simulink model "BaseEngineController_LS"  (Simulink 7.7)
settings: Solver=FixedStepDiscrete  StartTime=0.0  StopTime=10.0  RelTol=1e-3
PreLoadFcn:
  | try, eval([bdroot '_setup']); catch, eval('model_setup', ''); end
InitFcn:
  | try, eval([bdroot '_setup']); catch, eval('model_setup', ''); end
undefined symbols (not defined in the file): ECU555, High, motohawk_build_version, motohawk_trunc_name, motohawk_vardec_config_group, motohawk_vardec_path, True
libraries: MotoHawk_lib x1418, motohawk_control_primitives_lib x183, motohawk_engine_lib x32, simulink x21, motohawk_annotations_lib x9, AutoDoc_lib x8, simulink_extras x4, motohawk_ccp_examples_lib x1, motohawk_control_primitives_motoshare_lib x1
(part 21 of 27)

== system BaseEngineController_LS/Foreground/Control/Controller/Run/Fuel System Manager/O2 Fuel Adapt ==
  O2 Info : Inport
  Sensors : Inport  Port=2
  Abs : Abs  SaturateOnIntegerOverflow=on
  Adapt FuelFlowComp Map Bank A : Subsystem  TreatAsAtomicUnit=on
  Adapt FuelFlowComp Map Bank B : Subsystem  TreatAsAtomicUnit=on
  Bus Selector1 : BusSelector  OutputSignals=O2Error.O2ITerm_BankA
  Bus Selector2 : BusSelector  OutputSignals=O2ControlEnable.BankAEnable
  Bus Selector3 : BusSelector  OutputSignals=RawIndexes.MAP09Idx,RawIndexes.RPM09Idx
  Bus Selector4 : BusSelector  OutputSignals=DesiredLambda.WarmUpRatio,DesiredLambda.WarmUptimeRatio,DesiredLambda.DesEquivRatio
  Bus Selector5 : BusSelector  OutputSignals=O2Error.O2ITerm_BankB
  Divide : Product  Inputs=**
  Divide1 : Product  Inputs=**
  Logical Operator2 : Logic  Inputs=5
  MinMax : MinMax  Function=max  Inputs=2
  O2 Control Enable Delay : Subsystem  TreatAsAtomicUnit=on
  Product0 : Product  SaturateOnIntegerOverflow=on  InputSameDT=on  OutDataTypeStr=Inherit: Same as first input
  Product1 : Product  SaturateOnIntegerOverflow=on  InputSameDT=on  OutDataTypeStr=Inherit: Same as first input
  Relational Operator : RelationalOperator  Operator=<=  InputSameDT=on
  Saturation (Tunable) : Subsystem  AncestorBlock=motohawk_control_primitives_lib/Saturation (Tunable)  mask(Saturation (Tunable)){prefix='FuelAdaptError_BankA', UprLim=1, LwrLim=-1, units='', grp=motohawk_vardec_path(gcb)}
      mask prompts: UprLim "Upper Limit"; LwrLim "Lower Limit"; grp "MotoTune Group String"
      mask help: Saturation block with calibratable min/max values.
      mask Display:
      | patch([0 0 1 1], [0 0.075 0.075 0], [230/255 0/255 0/255])
      | patch([0 0 1 1], [0.025 0.05 0.05 0.025], [150/255 0/255 0/255])
      | patch([0 0 1 1], [0 0.025 0.025 0], [0/255 0/255 0/255])
      | 
      | plot([0 .2 .8 1], [.1 .1 1 1])
  Saturation (Tunable)1 : Subsystem  AncestorBlock=motohawk_control_primitives_lib/Saturation (Tunable)  mask(Saturation (Tunable)){prefix='FuelAdaptError_BankB', UprLim=1, LwrLim=-1, units='', grp=motohawk_vardec_path(gcb)}
      mask prompts: UprLim "Upper Limit"; LwrLim "Lower Limit"; grp "MotoTune Group String"
      mask help: Saturation block with calibratable min/max values.
      mask Display:
      | patch([0 0 1 1], [0 0.075 0.075 0], [230/255 0/255 0/255])
      | patch([0 0 1 1], [0.025 0.05 0.05 0.025], [150/255 0/255 0/255])
      | patch([0 0 1 1], [0 0.025 0.025 0], [0/255 0/255 0/255])
      | 
      | plot([0 .2 .8 1], [.1 .1 1 1])
  WarmUp Disable : Subsystem  TreatAsAtomicUnit=on
  motohawk_calibration : MotoHawk_lib/Calibration & Probing Blocks/motohawk_calibration  nam='AdaptEnable'  val=true  storage=Calibration  show_more=on  name_source=Use Parameter  data_type=Inherit from 'Default Value'  read_level=1  write_level=1  ovr_cals=on  view_as=Enumeration  enum_struct={'Disabled', 'Enabled'}  vector_style=Wide Row  use_help_units=on  help='Determines whether the FuelFlowComp map will be adapted using the MAF sensor'  units='bool'  use_header_enum=off  row_header_enum={}  col_header_enum={}  use_min_max=off  min_val=-inf  max_val=inf  use_precision=off  precision=''  gain=1  offset=0  exp=1  use_mototune_group=on  mototune_group=motohawk_vardec_path(gcb)
  motohawk_calibration1 : MotoHawk_lib/Calibration & Probing Blocks/motohawk_calibration  nam='FuelAdaptDelta'  val=0.5  storage=Calibration  show_more=on  name_source=Use Parameter  data_type=Inherit from 'Default Value'  read_level=1  write_level=1  ovr_cals=on  view_as=Number  enum_struct={'Disabled', 'Enabled'}  vector_style=Wide Row  use_help_units=on  help='O2_Error must be less than this delta to adapt the FuelFlowComp map'  units='mult'  use_header_enum=off  row_header_enum={}  col_header_enum={}  use_min_max=on  min_val=0  max_val=2  use_precision=off  precision=''  gain=1  offset=0  exp=1  use_mototune_group=on  mototune_group=motohawk_vardec_path(gcb)
  motohawk_calibration2 : MotoHawk_lib/Calibration & Probing Blocks/motohawk_calibration  nam='FuelAdaptEnable'  val=false  storage=Calibration  show_more=on  name_source=Use Parameter  data_type=Inherit from 'Default Value'  read_level=1  write_level=1  ovr_cals=on  view_as=Enumeration  enum_struct={'Disabled', 'Enabled'}  vector_style=Wide Row  use_help_units=on  help='Determines whether the FuelFlowComp map will be adapted using the MAF sensor'  units='bool'  use_header_enum=off  row_header_enum={}  col_header_enum={}  use_min_max=off  min_val=-inf  max_val=inf  use_precision=off  precision=''  gain=1  offset=0  exp=1  use_mototune_group=on  mototune_group=motohawk_vardec_path(gcb)
  motohawk_interpolation_1d1 : MotoHawk_lib/Lookup Tables/motohawk_interpolation_1d  nam='FuelAdaptGain_BankA'  table_data=[0,0,0,0,0]  show_more=on  data_type=Inherit from 'Table Data'  storage=NonAdaptive  read_level=1  write_level=1  ovr_cals=on  use_help=on  help="'Gain for updating FuelFlowComp map.  This fraction of the error is added to the map every 5ms.'"  units=''  use_min_max=off  min_val=-inf  max_val=inf  use_precision=on  precision='1.4'  gain=1  offset=0  exp=1  use_links=off  prelookup_block=''  output_name=''  use_mototune_group=on  mototune_group=motohawk_vardec_path(gcb)
  motohawk_interpolation_1d2 : MotoHawk_lib/Lookup Tables/motohawk_interpolation_1d  nam='FuelAdaptGain_BankB'  table_data=[0,0,0,0,0]  show_more=on  data_type=Inherit from 'Table Data'  storage=NonAdaptive  read_level=1  write_level=1  ovr_cals=on  use_help=on  help="'Gain for updating FuelFlowComp map.  This fraction of the error is added to the map every 5ms.'"  units=''  use_min_max=off  min_val=-inf  max_val=inf  use_precision=on  precision='1.4'  gain=1  offset=0  exp=1  use_links=off  prelookup_block=''  output_name=''  use_mototune_group=on  mototune_group=motohawk_vardec_path(gcb)
  motohawk_interpolation_2d1 : MotoHawk_lib/Lookup Tables/motohawk_interpolation_2d  nam='FuelFlowComp'  table_data=ones(9)  show_more=on  data_type=Inherit from 'Table Data'  storage=NonAdaptive  read_level=1  write_level=1  ovr_cals=on  use_help=on  help='Fuel Flow Compensation Multiplier - gain to adjust modelling errors in mechanical fuel system.'  units='mult'  use_min_max=on  min_val=-inf  max_val=inf  use_precision=on  precision=''  gain=1  offset=0  exp=1  use_links=off  row_prelookup_block=''  col_prelookup_block=''  output_name=''  use_mototune_group=on  mototune_group=motohawk_vardec_path(gcb)
  motohawk_interpolation_2d2 : MotoHawk_lib/Lookup Tables/motohawk_interpolation_2d  nam='FuelFlowCompAdapt_BankA'  table_data=ones(9)  show_more=on  data_type=Inherit from 'Table Data'  storage=Adaptive - NonVolatile  read_level=1  write_level=1  ovr_cals=on  use_help=on  help='Adapt map based on O2 ITerm that is multiplied into FuelFlowComp.'  units='mult'  use_min_max=on  min_val=-inf  max_val=inf  use_precision=on  precision=''  gain=1  offset=0  exp=1  use_links=off  row_prelookup_block=''  col_prelookup_block=''  output_name=''  use_mototune_group=on  mototune_group=motohawk_vardec_path(gcb)
  motohawk_interpolation_2d3 : MotoHawk_lib/Lookup Tables/motohawk_interpolation_2d  nam='FuelFlowCompAdapt_BankB'  table_data=ones(9)  show_more=on  data_type=Inherit from 'Table Data'  storage=Adaptive - NonVolatile  read_level=1  write_level=1  ovr_cals=on  use_help=on  help='Adapt map based on O2 ITerm that is multiplied into FuelFlowComp.'  units='mult'  use_min_max=on  min_val=-inf  max_val=inf  use_precision=on  precision=''  gain=1  offset=0  exp=1  use_links=off  row_prelookup_block=''  col_prelookup_block=''  output_name=''  use_mototune_group=on  mototune_group=motohawk_vardec_path(gcb)
  motohawk_prelookup1 : MotoHawk_lib/Lookup Tables/motohawk_prelookup  nam='O2ITerm_BankB'  breakpoint_data=[0,0,0,0,0]  show_more=on  data_type=Inherit from 'Table Data'  storage=Constant  read_level=1  write_level=1  ovr_cals=on  use_help=on  help='Index for O2 ITerm.'  units='mult'  use_min_max=off  min_val=-inf  max_val=inf  use_precision=off  precision=''  gain=1  offset=0  exp=1  use_links=on  input_name=''  use_mototune_group=on  mototune_group=motohawk_vardec_path(gcb)
  motohawk_prelookup13 : MotoHawk_lib/Lookup Tables/motohawk_prelookup  nam='O2ITerm_BankA'  breakpoint_data=[0,0,0,0,0]  show_more=on  data_type=Inherit from 'Table Data'  storage=Constant  read_level=1  write_level=1  ovr_cals=on  use_help=on  help='Index for O2 ITerm.'  units='mult'  use_min_max=off  min_val=-inf  max_val=inf  use_precision=off  precision=''  gain=1  offset=0  exp=1  use_links=on  input_name=''  use_mototune_group=on  mototune_group=motohawk_vardec_path(gcb)
  motohawk_probe1 : MotoHawk_lib/Calibration & Probing Blocks/motohawk_probe  nam='FuelAdapt_Error_BankB'  show_more=on  name_source=Use Parameter  read_level=1  view_as=Number  enum_struct={'Disabled', 'Enabled'}  vector_style=Wide Row  use_help_units=on  help='Error in fuel flow at the current operating point, as compared to O2 sensor'  units=''  use_header_enum=off  row_header_enum={}  col_header_enum={}  use_precision=off  precision=''  gain=1  offset=0  exp=1  use_mototune_group=on  mototune_group=motohawk_vardec_path(gcb)
  motohawk_probe3 : MotoHawk_lib/Calibration & Probing Blocks/motohawk_probe  nam='FuelAdaptEnabled'  show_more=on  name_source=Use Parameter  read_level=1  view_as=Enumeration  enum_struct={'Not Enabled', 'Enabled'}  vector_style=Wide Row  use_help_units=on  help='Indicates whether FuelFlowComp map adapting is enabled'  units=''  use_header_enum=off  row_header_enum={}  col_header_enum={}  use_precision=off  precision=''  gain=1  offset=0  exp=1  use_mototune_group=on  mototune_group=motohawk_vardec_path(gcb)
  motohawk_probe7 : MotoHawk_lib/Calibration & Probing Blocks/motohawk_probe  nam='FuelAdapt_Error_BankA'  show_more=on  name_source=Use Parameter  read_level=1  view_as=Number  enum_struct={'Disabled', 'Enabled'}  vector_style=Wide Row  use_help_units=on  help='Error in fuel flow at the current operating point, as compared to O2 sensor'  units=''  use_header_enum=off  row_header_enum={}  col_header_enum={}  use_precision=off  precision=''  gain=1  offset=0  exp=1  use_mototune_group=on  mototune_group=motohawk_vardec_path(gcb)
  "Adapt Fuel Mult Bank A " : Outport
  Adapt Fuel Mult Bank B : Outport  Port=2
  wires:
  Abs/1 -> Relational Operator/1
  motohawk_calibration1/1 -> Relational Operator/2
  motohawk_interpolation_1d1/1 -> Product0/2
  Product0/1 -> Saturation (Tunable)/1(In)
  Sensors/1 -> Bus Selector3/1
  O2 Info/1 -> Bus Selector2/1, Bus Selector4/1, Bus Selector1/1, Bus Selector5/1
  Bus Selector1/1 -> motohawk_prelookup13/1, Product0/1, MinMax/1  "<O2ITerm_BankA>"
  Bus Selector2/1 -> O2 Control Enable Delay/1(State_In)  "<BankAEnable>"
  Relational Operator/1 -> Logical Operator2/5
  WarmUp Disable/1(State_Out) -> Logical Operator2/3
  O2 Control Enable Delay/1(State_Out) -> Logical Operator2/4
  Logical Operator2/1 -> Adapt FuelFlowComp Map Bank A/Enable, motohawk_probe3/1, Adapt FuelFlowComp Map Bank B/Enable
  Saturation (Tunable)/1(Out) -> Adapt FuelFlowComp Map Bank A/1(AdaptError), motohawk_probe7/1
  motohawk_calibration/1 -> Logical Operator2/2
  motohawk_calibration2/1 -> Logical Operator2/1
  motohawk_interpolation_2d1/1 -> Divide/1, Divide1/2
  Divide/1 -> "Adapt Fuel Mult Bank A "/1
  motohawk_interpolation_2d2/1 -> Adapt FuelFlowComp Map Bank A/2(Adapt), Divide/2
  Bus Selector3/1 -> motohawk_interpolation_2d2/1, motohawk_interpolation_2d1/1, motohawk_interpolation_2d3/1  "<MAP09Idx>"
  Bus Selector3/2 -> motohawk_interpolation_2d2/2, motohawk_interpolation_2d1/2, motohawk_interpolation_2d3/2  "<RPM09Idx>"
  Bus Selector4/3 -> WarmUp Disable/3(BaseRatio)  "<DesEquivRatio>"
  Bus Selector4/2 -> WarmUp Disable/2(WarmupTimeRatio)  "<WarmUptimeRatio>"
  Bus Selector4/1 -> WarmUp Disable/1(WarmupRatio)  "<WarmUpRatio>"
  motohawk_prelookup13/1 -> motohawk_interpolation_1d1/1
  motohawk_prelookup1/1 -> motohawk_interpolation_1d2/1
  Product1/1 -> Saturation (Tunable)1/1(In)
  Saturation (Tunable)1/1(Out) -> Adapt FuelFlowComp Map Bank B/1(AdaptError), motohawk_probe1/1
  motohawk_interpolation_1d2/1 -> Product1/2
  Bus Selector5/1 -> motohawk_prelookup1/1, Product1/1, MinMax/2  "<O2ITerm_BankB>"
  motohawk_interpolation_2d3/1 -> Divide1/1, Adapt FuelFlowComp Map Bank B/2(Adapt)
  Divide1/1 -> Adapt Fuel Mult Bank B/1
  MinMax/1 -> Abs/1

== system BaseEngineController_LS/Foreground/Control/Controller/Run/MaxGovernor/I-Term Preload ==
  TotalETCReq : Inport
  RPMAccelIdx : Inport  Port=2
  Sum : Sum  Inputs=|+-
  motohawk_interpolation_1d4 : MotoHawk_lib/Lookup Tables/motohawk_interpolation_1d  nam='MaxGovPreloadITerm'  table_data=[1 30 50 51.18 52.349998 53.529999 54.709999 55.880001 57.060001 58.240002 59.41 60.59 61.759998 62.939999 67.650002 68.82 70]  show_more=on  data_type=Inherit from 'Table Data'  storage=NonAdaptive  read_level=1  write_level=1  ovr_cals=on  use_help=on  help='Preload for Max Gov PID ITerm based on engine acceleration rate upon entry into max gov.'  units='%'  use_min_max=on  min_val=-inf  max_val=inf  use_precision=on  precision=''  gain=1  offset=0  exp=1  use_links=off  prelookup_block=''  output_name=''  use_mototune_group=on  mototune_group=motohawk_vardec_path(gcb)
  motohawk_probe : MotoHawk_lib/Calibration & Probing Blocks/motohawk_probe  nam='MaxGovIC'  show_more=on  name_source=Use Parameter  read_level=1  view_as=Number  enum_struct={'Disabled', 'Enabled'}  vector_style=Wide Row  use_help_units=off  help=''  units=''  use_header_enum=off  row_header_enum={}  col_header_enum={}  use_precision=off  precision=''  gain=1  offset=0  exp=1  use_mototune_group=on  mototune_group=motohawk_vardec_path(gcb)
  ITerm Preload : Outport
  wires:
  RPMAccelIdx/1 -> motohawk_interpolation_1d4/1
  Sum/1 -> ITerm Preload/1, motohawk_probe/1
  motohawk_interpolation_1d4/1 -> Sum/2
  TotalETCReq/1 -> Sum/1

== system BaseEngineController_LS/Foreground/Control/Controller/Run/MaxGovernor/MaxGovState ==
  note: Move into On State if RPM > EntryCriteria or Target.
      | Move into Trans State if APP falls below TPS, PID controller is frozen during Trans State, but output is based on APP.
      | 	When in AllSpeedGov mode, switch to Trans if AllSpeedGov setpoint is less than MaxGov setpoint minus hyst.
      | Move from Trans State back to On State if RPM > Target.
      | Move from Trans State to Off if RPM < Entry Criteria.
  RPMEntryCriteria : Inport
  TotalETCReq : Inport  Port=2
  Sensors : Inport  Port=3
  TargetRPM : Inport  Port=4
  Bus Selector : BusSelector  OutputSignals=RawProcessed.TPS
  Bus Selector1 : BusSelector  OutputSignals=Raw.RPMInst
  Constant : Constant  Value=boolean(0)
  Data Type Conversion : DataTypeConversion  OutDataTypeStr=int8
  Data Type Conversion1 : DataTypeConversion  OutDataTypeStr=int8
  Data Type Conversion2 : DataTypeConversion  OutDataTypeStr=int8
  Logical Operator : Logic  Operator=NOT  AllPortsSameDT=off  OutDataTypeStr=boolean
  Logical Operator1 : Logic  AllPortsSameDT=off  OutDataTypeStr=boolean
  Logical Operator2 : Logic  Operator=OR  AllPortsSameDT=off  OutDataTypeStr=boolean
  Logical Operator3 : Logic  Operator=OR  AllPortsSameDT=off  OutDataTypeStr=boolean
  MaxGOV Stateflow : Stateflow chart  TreatAsAtomicUnit=on
  Multiport Switch : MultiPortSwitch  DataPortOrder=Zero-based contiguous  Inputs=2  zeroidx=on
  Relational Operator : RelationalOperator  Operator=<=  OutDataTypeStr=boolean
  Relational Operator1 : RelationalOperator  Operator=>  OutDataTypeStr=boolean
  Relational Operator2 : RelationalOperator  Operator=>  OutDataTypeStr=boolean
  Sum : Sum  Inputs=|+-
  Sum1 : Sum  Inputs=++|
  motohawk_calibration1 : MotoHawk_lib/Calibration & Probing Blocks/motohawk_calibration  nam='MaxGovDisable'  val=0  storage=Calibration  show_more=on  name_source=Use Parameter  data_type=boolean  read_level=1  write_level=1  ovr_cals=on  view_as=Enumeration  enum_struct={'Gov Enabled', 'Gov Disabled'}  vector_style=Wide Row  use_help_units=on  help='Max governor manual disable'  units=''  use_header_enum=off  row_header_enum={}  col_header_enum={}  use_min_max=off  min_val=0  max_val=inf  use_precision=off  precision=''  gain=1  offset=0  exp=1  use_mototune_group=on  mototune_group=motohawk_vardec_path(gcb)
  motohawk_calibration5 : MotoHawk_lib/Calibration & Probing Blocks/motohawk_calibration  nam='MaxGovTPSHyst'  val=4  storage=Calibration  show_more=on  name_source=Use Parameter  data_type=Inherit from 'Default Value'  read_level=1  write_level=1  ovr_cals=on  view_as=Number  enum_struct={'Disabled', 'Enabled'}  vector_style=Wide Row  use_help_units=on  help='Hysterisis around max gov TPS entry criteria.'  units='%'  use_header_enum=off  row_header_enum={}  col_header_enum={}  use_min_max=on  min_val=0  max_val=inf  use_precision=on  precision=''  gain=1  offset=0  exp=1  use_mototune_group=on  mototune_group=motohawk_vardec_path(gcb)
  motohawk_data_def : MotoHawk_lib/Data Storage Blocks/motohawk_data_def  nam='MaxGov'  container_nam=''  data=0  typ=double  struct_nam='MyStruct'  storage=Volatile  outputRef=off  use_vardec=off  window=Display  read_level=1  write_level=1  ovr_cals=on  view_as=Number  enum_struct={'Disabled', 'Enabled'}  vector_style=Wide Row  use_help_units=off  help=''  units=''  use_header_enum=off  row_header_enum=''  col_header_enum=''  use_min_max=off  min_val=-inf  max_val=inf  use_precision=off  precision=''  gain=1  offset=0  exp=1  use_mototune_group=off  mototune_group=motohawk_vardec_path(gcb)  eval_name=MyData  data_stores=motohawk_sfun_data_def_data_stores  struct_instances=motohawk_sfun_data_def_struct_instances  vardecs=motohawk_sfun_data_def_vardecs
  motohawk_data_read : MotoHawk_lib/Data Storage Blocks/motohawk_data_read  source=Lookup By Name  structure=Scalar  operation=Read scalar from location by index  sz_vec=4  sz_row=2  sz_col=3  typ=double  nam='MaxGov'  checkNull=on  struct_inst_name='MyData'  struct_nam='MyStruct'
  motohawk_data_write : MotoHawk_lib/Data Storage Blocks/motohawk_data_write  source=Lookup By Name  structure=Scalar  operation=Write entire data structure at once  sz_vec=9  sz_row=2  sz_col=9  typ=double  nam='MaxGov'  checkNull=on  write_read_only=off  struct_inst_name=''  struct_name='MyStruct'
  motohawk_probe : MotoHawk_lib/Calibration & Probing Blocks/motohawk_probe  nam='MaxGovETCMode'  show_more=on  name_source=Use Parameter  read_level=1  view_as=Enumeration  enum_struct={'ETC Req Mode','PID Mode'}  vector_style=Wide Row  use_help_units=on  help=''  units=''  use_header_enum=off  row_header_enum={}  col_header_enum={}  use_precision=on  precision=''  gain=1  offset=0  exp=1  use_mototune_group=on  mototune_group=motohawk_vardec_path(gcb)
  motohawk_probe1 : MotoHawk_lib/Calibration & Probing Blocks/motohawk_probe  nam='MaxGovHold'  show_more=on  name_source=Use Parameter  read_level=1  view_as=Enumeration  enum_struct={'Hold Off','Hold On'}  vector_style=Wide Row  use_help_units=on  help=''  units=''  use_header_enum=off  row_header_enum={}  col_header_enum={}  use_precision=on  precision=''  gain=1  offset=0  exp=1  use_mototune_group=on  mototune_group=motohawk_vardec_path(gcb)
  motohawk_probe2 : MotoHawk_lib/Calibration & Probing Blocks/motohawk_probe  nam='MaxGovReset'  show_more=on  name_source=Use Parameter  read_level=1  view_as=Enumeration  enum_struct={'Reset Off','Reset On'}  vector_style=Wide Row  use_help_units=on  help=''  units=''  use_header_enum=off  row_header_enum={}  col_header_enum={}  use_precision=on  precision=''  gain=1  offset=0  exp=1  use_mototune_group=on  mototune_group=motohawk_vardec_path(gcb)
  motohawk_probe4 : MotoHawk_lib/Calibration & Probing Blocks/motohawk_probe  nam='MaxGovState'  show_more=on  name_source=Use Parameter  read_level=1  view_as=Enumeration  enum_struct={'Disabled', 'Enabled'}  vector_style=Wide Row  use_help_units=off  help=''  units=''  use_header_enum=off  row_header_enum={}  col_header_enum={}  use_precision=off  precision=''  gain=1  offset=0  exp=1  use_mototune_group=on  mototune_group=motohawk_vardec_path(gcb)
  ETCMode : Outport
  PIDReset : Outport  Port=2
  PIDHold : Outport  Port=3
  wires:
  Relational Operator/1 -> MaxGOV Stateflow/2(OnToTrans)
  motohawk_calibration5/1 -> Sum/2, Sum1/1
  Sensors/1 -> Bus Selector/1, Bus Selector1/1
  Bus Selector/1 -> Sum/1, Sum1/2  "<TPS>"
  Sum/1 -> Relational Operator/2
  Sum1/1 -> Relational Operator1/2
  TotalETCReq/1 -> Relational Operator/1, Relational Operator1/1
  RPMEntryCriteria/1 -> Logical Operator1/1, Logical Operator/1, Logical Operator3/1
  Relational Operator1/1 -> Logical Operator1/2
  MaxGOV Stateflow/3(Hold) -> Data Type Conversion1/1
  Logical Operator/1 -> MaxGOV Stateflow/4(TransToOff)
  Bus Selector1/1 -> Relational Operator2/1  "<RPMInst>"
  TargetRPM/1 -> Relational Operator2/2
  Logical Operator2/1 -> MaxGOV Stateflow/3(TransToOn)
  Logical Operator1/1 -> Logical Operator2/1
  Relational Operator2/1 -> Logical Operator2/2, Logical Operator3/2
  MaxGOV Stateflow/2(Reset) -> Data Type Conversion/1
  Logical Operator3/1 -> MaxGOV Stateflow/1(OffToOn)
  MaxGOV Stateflow/1(ETCMode) -> Data Type Conversion2/1
  Multiport Switch/1 -> ETCMode/1, motohawk_probe4/1, motohawk_probe/1
  Constant/1 -> Multiport Switch/3
  MaxGOV Stateflow/4(StateO) -> motohawk_data_write/1
  motohawk_data_read/1 -> MaxGOV Stateflow/5(State)
  Data Type Conversion/1 -> PIDReset/1, motohawk_probe2/1
  Data Type Conversion1/1 -> PIDHold/1, motohawk_probe1/1
  Data Type Conversion2/1 -> Multiport Switch/2
  motohawk_calibration1/1 -> Multiport Switch/1

== system BaseEngineController_LS/Foreground/Control/Controller/Run/MaxGovernor/Ramp RPM ==
  note: 1st-Order Ramp Up
  note: y[k] = a*x[k] + (1-a)*y[k-1]
  note: where a = t/T
  OnIdle : Inport
  TargetRPM : Inport  Port=2
  RPM : Inport  Port=3
  Constant : Constant  OutDataTypeStr=Inherit: Inherit via back propagation
  Don't allow setpoint to ever go above the TargetRPM : MinMax  Inputs=2  SaturateOnIntegerOverflow=on  InputSameDT=on
  Logical Operator : Logic  Operator=NOT
  Preload lowpass filter with current RPM while not on Idle : Switch  Threshold=0.5  ZeroCross=off  SaturateOnIntegerOverflow=on  InputSameDT=on
  Product1 : Product  Inputs=*/  SaturateOnIntegerOverflow=on  InputSameDT=on  OutDataTypeStr=Inherit: Same as first input
  Product2 : Product  SaturateOnIntegerOverflow=on  InputSameDT=on  OutDataTypeStr=Inherit: Same as first input
  Product3 : Product  SaturateOnIntegerOverflow=on  InputSameDT=on  OutDataTypeStr=Inherit: Same as first input
  Sum : Sum  Inputs=-+|  SaturateOnIntegerOverflow=on
  Sum1 : Sum  SaturateOnIntegerOverflow=on
  Unit Delay : UnitDelay  SampleTime=-1
  motohawk_calibration2 : MotoHawk_lib/Calibration & Probing Blocks/motohawk_calibration  nam='MaxGovRPMCtrlEntryFiltC'  val=0.2  storage=Calibration  show_more=on  name_source=Use Parameter  data_type=Inherit from 'Default Value'  read_level=1  write_level=1  ovr_cals=on  view_as=Number  enum_struct={'Disabled', 'Enabled'}  vector_style=Wide Row  use_help_units=on  help='Filter rate at which Max Gov setup is increased to MaxGovBaseRPMSetpoint.'  units='sec'  use_header_enum=off  row_header_enum={}  col_header_enum={}  use_min_max=on  min_val=.005  max_val=inf  use_precision=off  precision=''  gain=1  offset=0  exp=1  use_mototune_group=on  mototune_group=motohawk_vardec_path(gcb)
  motohawk_delta_time : MotoHawk_lib/Extra Development Blocks/motohawk_delta_time  samp_time=-1  init_val=0  mode=Seconds (double)
  motohawk_probe3 : MotoHawk_lib/Calibration & Probing Blocks/motohawk_probe  nam='MaxGovRPMSetpoint'  show_more=on  name_source=Use Parameter  read_level=1  view_as=Number  enum_struct={'Disabled', 'Enabled'}  vector_style=Wide Row  use_help_units=on  help='RPMSetpoint of Max Gov controller.'  units='RPM'  use_header_enum=off  row_header_enum={}  col_header_enum={}  use_precision=on  precision=''  gain=1  offset=0  exp=1  use_mototune_group=on  mototune_group=motohawk_vardec_path(gcb)
  RPMSetPt : Outport
  wires:
  Logical Operator/1 -> Preload lowpass filter with current RPM while not on Idle/2
  Don't allow setpoint to ever go above the TargetRPM/1 -> RPMSetPt/1, Unit Delay/1, motohawk_probe3/1
  Preload lowpass filter with current RPM while not on Idle/1 -> Don't allow setpoint to ever go above the TargetRPM/2
  RPM/1 -> Preload lowpass filter with current RPM while not on Idle/1
  TargetRPM/1 -> Don't allow setpoint to ever go above the TargetRPM/1, Product2/1
  Product1/1 -> Sum/1, Product2/2  "alpha"
  Constant/1 -> Sum/2
  Product2/1 -> Sum1/1
  Product3/1 -> Sum1/2
  Sum/1 -> Product3/1
  Unit Delay/1 -> Product3/2
  motohawk_delta_time/1 -> Product1/1
  motohawk_calibration2/1 -> Product1/2
  Sum1/1 -> Preload lowpass filter with current RPM while not on Idle/3
  OnIdle/1 -> Logical Operator/1

== system BaseEngineController_LS/Foreground/Control/Controller/Run/MaxGovernor/Trigger Pre-load ==
  RPM : Inport
  GearState : Inport  Port=2
  InGear : Subsystem  TreatAsAtomicUnit=on
  InNeutral : Subsystem  TreatAsAtomicUnit=on
  Logical Operator : Logic  Operator=NOT  AllPortsSameDT=off  OutDataTypeStr=boolean
  Merge : Merge
  Merge1 : Merge
  Relational Operator : RelationalOperator  Operator=>  OutDataTypeStr=boolean
  Sum1 : Sum  Inputs=+-|
  Trigger : Outport
  BaseRPMSetpoint : Outport  Port=2
  wires:
  Relational Operator/1 -> Trigger/1
  RPM/1 -> Relational Operator/1
  Sum1/1 -> Relational Operator/2
  InGear/1(BaseSetpoint) -> Merge/1
  InGear/2(Threshold) -> Merge1/1
  InNeutral/1(BaseSetpoint) -> Merge/2
  InNeutral/2(Threshold) -> Merge1/2
  Merge/1 -> Sum1/1, BaseRPMSetpoint/1
  Merge1/1 -> Sum1/2
  GearState/1 -> InGear/Enable, Logical Operator/1
  Logical Operator/1 -> InNeutral/Enable

== system BaseEngineController_LS/Foreground/Control/Controller/Run/MaxGovernor/Universal PID (Tunable & Scheduled) ==
  ITerm IC : Inport
  Reset All : Inport  Port=2
  Hold PID : Inport  Port=3
  SetPoint : Inport  Port=4
  Actual : Inport  Port=5
  Constant : Constant  Value=0
  Product3 : Product  SaturateOnIntegerOverflow=on  InputSameDT=on  OutDataTypeStr=Inherit: Same as first input
  Product4 : Product  SaturateOnIntegerOverflow=on  InputSameDT=on  OutDataTypeStr=Inherit: Same as first input
  Product5 : Product  SaturateOnIntegerOverflow=on  InputSameDT=on  OutDataTypeStr=Inherit: Same as first input
  Saturation : motohawk_control_primitives_lib/Saturation  SystemSampleTime=-1
  Switch : Switch  Threshold=1
  Switch1 : Switch  Threshold=1
  Universal PID : motohawk_control_primitives_lib/Universal PID  Description=|  SystemSampleTime=-1  samp_time=.005
      | /* Name: ErrorGain Unit:mult ClassID:VAR StorageID:FLASH Access:RW4+RW3+NA2+NA1 TypeID:UINT4                   
      |    Gain:0.000000001 Min:0.000000000 Max:4.000000000 Format:10.9 UpdateID:REMOTE Help:"This gain is applied to "
      |    "the error term before it is used to calculate the P, I and D terms." VardecSig:6C */                       
      |                                                                                                                
      | /* Name: ITermLowerLim Unit:0 ClassID:VAR StorageID:FLASH Access:RW4+RW3+NA2+NA1 TypeID:SINT2 Gain:0.1         
      |    Min:-3276.8 Max:3276.7 Format:5.1 UpdateID:REMOTE Help:"Lower limit on the I-term value." VardecSig:6C */   
      |                                                                                                                
      | /* Name: ITermUpperLim ClassID:VAR StorageID:FLASH Access:RW4+RW3+NA2+NA1 TypeID:SINT2 Gain:0.1 Min:-3276.8    
      |    Max:3276.7 Format:5.1 UpdateID:REMOTE Help:"Upper limit on I-term value." VardecSig:6C */                   
      |                                                                                                                
      | /* Name: PIDOutLowerLim ClassID:VAR StorageID:FLASH Access:RW4+RW3+NA2+NA1 TypeID:SINT2 Gain:0.1               
      |    Min:-3276.8 Max:3276.7 Format:5.1 UpdateID:REMOTE Help:"Lower limit on PID output." VardecSig:6C */         
      |                                                                                                                
      | /* Name: PIDOutUpperLim ClassID:VAR StorageID:FLASH Access:RW4+RW3+NA2+NA1 TypeID:SINT2 Gain:0.1               
      |    Min:-3276.8 Max:3276.7 Format:3.1 UpdateID:REMOTE Help:"Upper limit on PID output." VardecSig:6C */
  motohawk_calibration2 : MotoHawk_lib/Calibration & Probing Blocks/motohawk_calibration  nam=[prefix 'PIDOutUpperLimit']  val=100  storage=Calibration  show_more=on  name_source=Use Parameter  data_type=Inherit from 'Default Value'  read_level=1  write_level=1  ovr_cals=on  view_as=Number  enum_struct={'Disabled', 'Enabled'}  vector_style=Wide Row  use_help_units=on  help='Upper limit on max governor PID Output.'  units='%'  use_header_enum=off  row_header_enum={}  col_header_enum={}  use_min_max=on  min_val=-inf  max_val=inf  use_precision=on  precision=''  gain=1  offset=0  exp=1  use_mototune_group=on  mototune_group=motohawk_vardec_path(gcb)
  motohawk_calibration3 : MotoHawk_lib/Calibration & Probing Blocks/motohawk_calibration  nam=[prefix 'PGain']  val=0.5  storage=Calibration  show_more=on  name_source=Use Parameter  data_type=Inherit from 'Default Value'  read_level=1  write_level=1  ovr_cals=on  view_as=Number  enum_struct={'Disabled', 'Enabled'}  vector_style=Wide Row  use_help_units=on  help='Base P-gain for the max. governor controller.'  units='mult'  use_header_enum=off  row_header_enum={}  col_header_enum={}  use_min_max=off  min_val=-inf  max_val=inf  use_precision=off  precision=''  gain=1  offset=0  exp=1  use_mototune_group=on  mototune_group=motohawk_vardec_path(gcb)
  motohawk_calibration4 : MotoHawk_lib/Calibration & Probing Blocks/motohawk_calibration  nam=[prefix 'IGain']  val=1  storage=Calibration  show_more=on  name_source=Use Parameter  data_type=Inherit from 'Default Value'  read_level=1  write_level=1  ovr_cals=on  view_as=Number  enum_struct={'Disabled', 'Enabled'}  vector_style=Wide Row  use_help_units=on  help='Base I-gain for the max. governor controller.'  units='mult'  use_header_enum=off  row_header_enum={}  col_header_enum={}  use_min_max=off  min_val=-inf  max_val=inf  use_precision=off  precision=''  gain=1  offset=0  exp=1  use_mototune_group=on  mototune_group=motohawk_vardec_path(gcb)
  motohawk_calibration5 : MotoHawk_lib/Calibration & Probing Blocks/motohawk_calibration  nam=[prefix 'ErrorGain']  val=0.1  storage=Calibration  show_more=on  name_source=Use Parameter  data_type=Inherit from 'Default Value'  read_level=1  write_level=1  ovr_cals=on  view_as=Number  enum_struct={'Disabled', 'Enabled'}  vector_style=Wide Row  use_help_units=on  help='Error gain for the max governor controller. This gain is applied to the RPM error term before it is used to calculate the P, I and D terms.'  units='mult'  use_header_enum=off  row_header_enum={}  col_header_enum={}  use_min_max=on  min_val=-inf  max_val=inf  use_precision=off  precision=''  gain=1  offset=0  exp=1  use_mototune_group=on  mototune_group=motohawk_vardec_path(gcb)
  motohawk_calibration6 : MotoHawk_lib/Calibration & Probing Blocks/motohawk_calibration  nam=[prefix 'DGain']  val=0  storage=Calibration  show_more=on  name_source=Use Parameter  data_type=Inherit from 'Default Value'  read_level=1  write_level=1  ovr_cals=on  view_as=Number  enum_struct={'Disabled', 'Enabled'}  vector_style=Wide Row  use_help_units=on  help='Base D-gain for the max. governor controller.'  units='mult'  use_header_enum=off  row_header_enum={}  col_header_enum={}  use_min_max=off  min_val=-inf  max_val=inf  use_precision=off  precision=''  gain=1  offset=0  exp=1  use_mototune_group=on  mototune_group=motohawk_vardec_path(gcb)
  motohawk_calibration7 : MotoHawk_lib/Calibration & Probing Blocks/motohawk_calibration  nam=[prefix 'ITermLowerLimit']  val=-10  storage=Calibration  show_more=on  name_source=Use Parameter  data_type=Inherit from 'Default Value'  read_level=1  write_level=1  ovr_cals=on  view_as=Number  enum_struct={'Disabled', 'Enabled'}  vector_style=Wide Row  use_help_units=on  help='Lower limit on max governor I-term value.'  units='%'  use_header_enum=off  row_header_enum={}  col_header_enum={}  use_min_max=off  min_val=-inf  max_val=inf  use_precision=off  precision=''  gain=1  offset=0  exp=1  use_mototune_group=on  mototune_group=motohawk_vardec_path(gcb)
  motohawk_calibration8 : MotoHawk_lib/Calibration & Probing Blocks/motohawk_calibration  nam=[prefix 'ITermUpperLimit']  val=100  storage=Calibration  show_more=on  name_source=Use Parameter  data_type=Inherit from 'Default Value'  read_level=1  write_level=1  ovr_cals=on  view_as=Number  enum_struct={'Disabled', 'Enabled'}  vector_style=Wide Row  use_help_units=on  help='Upper limit on max governor I-term value.'  units='%'  use_header_enum=off  row_header_enum={}  col_header_enum={}  use_min_max=off  min_val=-inf  max_val=inf  use_precision=off  precision=''  gain=1  offset=0  exp=1  use_mototune_group=on  mototune_group=motohawk_vardec_path(gcb)
  motohawk_calibration9 : MotoHawk_lib/Calibration & Probing Blocks/motohawk_calibration  nam=[prefix 'PIDOutLowerLimit']  val=-10  storage=Calibration  show_more=on  name_source=Use Parameter  data_type=Inherit from 'Default Value'  read_level=1  write_level=1  ovr_cals=on  view_as=Number  enum_struct={'Disabled', 'Enabled'}  vector_style=Wide Row  use_help_units=on  help='Lower limit on max governor PID Output.'  units='%'  use_header_enum=off  row_header_enum={}  col_header_enum={}  use_min_max=off  min_val=-inf  max_val=inf  use_precision=off  precision=''  gain=1  offset=0  exp=1  use_mototune_group=on  mototune_group=motohawk_vardec_path(gcb)
  motohawk_interpolation_1d2 : MotoHawk_lib/Lookup Tables/motohawk_interpolation_1d  nam=[prefix 'DGainErrorMult']  table_data=[0.01 0.055 0.1 0.1 0.1 0.1 0.1 0.1 0.1]  show_more=on  data_type=Inherit from 'Table Data'  storage=NonAdaptive  read_level=1  write_level=1  ovr_cals=on  use_help=on  help=''  units='mult'  use_min_max=off  min_val=-inf  max_val=inf  use_precision=off  precision=''  gain=1  offset=0  exp=1  use_links=off  prelookup_block=''  output_name=''  use_mototune_group=on  mototune_group=motohawk_vardec_path(gcb)
  motohawk_interpolation_1d3 : MotoHawk_lib/Lookup Tables/motohawk_interpolation_1d  nam=[prefix 'PGainErrorMult']  table_data=[2 1.67 1.33 1 1 1 1 1 1]  show_more=on  data_type=Inherit from 'Table Data'  storage=NonAdaptive  read_level=1  write_level=1  ovr_cals=on  use_help=on  help=''  units='mult'  use_min_max=on  min_val=-inf  max_val=inf  use_precision=on  precision=''  gain=1  offset=0  exp=1  use_links=off  prelookup_block=''  output_name=''  use_mototune_group=on  mototune_group=motohawk_vardec_path(gcb)
  motohawk_interpolation_1d4 : MotoHawk_lib/Lookup Tables/motohawk_interpolation_1d  nam=[prefix 'IGainErrorMult']  table_data=[15 7 4 1.7 1.6 1.6 2.2 2.8 3.4]  show_more=on  data_type=Inherit from 'Table Data'  storage=NonAdaptive  read_level=1  write_level=1  ovr_cals=on  use_help=on  help=''  units='mult'  use_min_max=on  min_val=-inf  max_val=inf  use_precision=off  precision=''  gain=1  offset=0  exp=1  use_links=off  prelookup_block=''  output_name=''  use_mototune_group=on  mototune_group=motohawk_vardec_path(gcb)
  motohawk_prelookup1 : MotoHawk_lib/Lookup Tables/motohawk_prelookup  nam=[prefix 'SpeedError']  breakpoint_data="[-100 -77.777779 -55.555557 -33.333332 -11.111111 11.111111  55.555557 77.777779 100]"  show_more=on  data_type=Inherit from 'Table Data'  storage=Constant  read_level=1  write_level=1  ovr_cals=on  use_help=on  help=''  units='RPM'  use_min_max=off  min_val=-inf  max_val=inf  use_precision=on  precision=''  gain=1  offset=0  exp=1  use_links=off  input_name=''  use_mototune_group=on  mototune_group=motohawk_vardec_path(gcb)
  motohawk_probe1 : MotoHawk_lib/Calibration & Probing Blocks/motohawk_probe  nam=[prefix 'PTerm']  show_more=on  name_source=Use Parameter  read_level=1  view_as=Number  enum_struct={'Disabled', 'Enabled'}  vector_style=Wide Row  use_help_units=on  help=''  units=''  use_header_enum=off  row_header_enum={}  col_header_enum={}  use_precision=on  precision=''  gain=1  offset=0  exp=1  use_mototune_group=on  mototune_group=motohawk_vardec_path(gcb)
  motohawk_probe2 : MotoHawk_lib/Calibration & Probing Blocks/motohawk_probe  nam=[prefix 'ITerm']  show_more=on  name_source=Use Parameter  read_level=1  view_as=Number  enum_struct={'Disabled', 'Enabled'}  vector_style=Wide Row  use_help_units=on  help=''  units=''  use_header_enum=off  row_header_enum={}  col_header_enum={}  use_precision=on  precision=''  gain=1  offset=0  exp=1  use_mototune_group=on  mototune_group=motohawk_vardec_path(gcb)
  motohawk_probe3 : MotoHawk_lib/Calibration & Probing Blocks/motohawk_probe  nam=[prefix 'DTerm']  show_more=on  name_source=Use Parameter  read_level=1  view_as=Number  enum_struct={'Disabled', 'Enabled'}  vector_style=Wide Row  use_help_units=on  help=''  units=''  use_header_enum=off  row_header_enum={}  col_header_enum={}  use_precision=on  precision=''  gain=1  offset=0  exp=1  use_mototune_group=on  mototune_group=motohawk_vardec_path(gcb)
  motohawk_probe6 : MotoHawk_lib/Calibration & Probing Blocks/motohawk_probe  nam=[prefix 'Error']  show_more=on  name_source=Use Parameter  read_level=1  view_as=Number  enum_struct={'Disabled', 'Enabled'}  vector_style=Wide Row  use_help_units=on  help=''  units=''  use_header_enum=off  row_header_enum={}  col_header_enum={}  use_precision=on  precision=''  gain=1  offset=0  exp=1  use_mototune_group=on  mototune_group=motohawk_vardec_path(gcb)
  MaxGovOut : Outport
  MaxGovITerm : Outport  Port=2
  wires:
  motohawk_interpolation_1d2/1 -> Product3/2
  motohawk_interpolation_1d3/1 -> Product4/2
  motohawk_calibration6/1 -> Product3/1
  Product3/1 -> Universal PID/6
  motohawk_calibration3/1 -> Product4/1
  Product4/1 -> Universal PID/4
  motohawk_calibration5/1 -> Universal PID/3
  Universal PID/1 -> Saturation/1
  Universal PID/5 -> motohawk_probe3/1
  SetPoint/1 -> Universal PID/2, Switch1/1
  motohawk_prelookup1/1 -> motohawk_interpolation_1d4/1, motohawk_interpolation_1d2/1, motohawk_interpolation_1d3/1
  motohawk_calibration4/1 -> Product5/1
  motohawk_interpolation_1d4/1 -> Product5/2
  Product5/1 -> Universal PID/5
  Universal PID/2 -> motohawk_prelookup1/1, motohawk_probe6/1
  Universal PID/3 -> motohawk_probe1/1
  Universal PID/4 -> motohawk_probe2/1, MaxGovITerm/1
  ITerm IC/1 -> Universal PID/7
  motohawk_calibration7/1 -> Universal PID/8
  motohawk_calibration8/1 -> Universal PID/9
  motohawk_calibration2/1 -> Saturation/3
  motohawk_calibration9/1 -> Saturation/2
  Reset All/1 -> Universal PID/10, Switch/2
  Saturation/1 -> Switch/3
  Constant/1 -> Switch/1
  Switch1/1 -> Universal PID/1
  Actual/1 -> Switch1/3
  Hold PID/1 -> Switch1/2
  Switch/1 -> MaxGovOut/1

== system BaseEngineController_LS/Foreground/Control/Controller/Run/MinGovernor/AiflowOffset ==
  Sensors : Inport
  AC : Inport  Port=2
  Bus Selector1 : BusSelector  OutputSignals=RawProcessed.TPS
  Bus Selector2 : BusSelector  OutputSignals=RawIndexes.ECT05Idx
  Bus Selector3 : BusSelector  OutputSignals=RawIndexes.ACPres05Idx
  Logical Operator : Logic  Operator=OR  AllPortsSameDT=off  OutDataTypeStr=boolean
  Product : Product  Inputs=3  RndMeth=Zero
  Ramp Air Into Idle State : Subsystem
      mask Display: disp('RAMP AIR\nINTO IDLE STATE');
  Relational Operator : RelationalOperator  Operator===  OutDataTypeStr=boolean
  Relational Operator1 : RelationalOperator  Operator=<  OutDataTypeStr=boolean
  Run : motohawk_control_primitives_lib/CompareTo  SystemSampleTime=-1  op===  val=3
  Sum : Sum
  Unit Delay : UnitDelay  SampleTime=-1
  motohawk_calibration : MotoHawk_lib/Calibration & Probing Blocks/motohawk_calibration  nam='ACAirFlowOfst_Enab'  val=0  storage=Calibration  show_more=on  name_source=Use Parameter  data_type=boolean  read_level=1  write_level=1  ovr_cals=on  view_as=Enumeration  enum_struct={'Disabled', 'Enabled'}  vector_style=Wide Row  use_help_units=on  help='Enables AC airflow adder'  units=''  use_header_enum=off  row_header_enum={}  col_header_enum={}  use_min_max=off  min_val=-inf  max_val=inf  use_precision=off  precision=''  gain=1  offset=0  exp=1  use_mototune_group=off  mototune_group=motohawk_vardec_path(gcb)
  motohawk_data_read : MotoHawk_lib/Data Storage Blocks/motohawk_data_read  source=Lookup By Name  structure=Scalar  operation=Read entire data structure at once  sz_vec=4  sz_row=2  sz_col=3  typ=uint8  nam='EngineState'  checkNull=on  struct_inst_name='Struct1'  struct_nam='MyStruct'
  motohawk_interpolation_1d1 : MotoHawk_lib/Lookup Tables/motohawk_interpolation_1d  nam='ACAirFlowOfst'  table_data=[1 1 1 1 1]  show_more=on  data_type=Inherit from 'Table Data'  storage=NonAdaptive  read_level=1  write_level=1  ovr_cals=on  use_help=on  help='AC air position in based on ECT.'  units='%'  use_min_max=on  min_val=-inf  max_val=inf  use_precision=on  precision=''  gain=1  offset=0  exp=1  use_links=off  prelookup_block=''  output_name=''  use_mototune_group=on  mototune_group=motohawk_vardec_path(gcb)
  motohawk_interpolation_1d2 : MotoHawk_lib/Lookup Tables/motohawk_interpolation_1d  nam='BaseAirflowOfst'  table_data=[1 1 1 1 1]  show_more=on  data_type=Inherit from 'Table Data'  storage=Adaptive - NonVolatile  read_level=1  write_level=1  ovr_cals=on  use_help=on  help='Base air position in based on ECT.'  units='%'  use_min_max=on  min_val=-inf  max_val=inf  use_precision=on  precision=''  gain=1  offset=0  exp=1  use_links=off  prelookup_block=''  output_name=''  use_mototune_group=on  mototune_group=motohawk_vardec_path(gcb)
  motohawk_probe1 : MotoHawk_lib/Calibration & Probing Blocks/motohawk_probe  nam='BaseAirOffset'  show_more=on  name_source=Use Parameter  read_level=1  view_as=Number  enum_struct={'Disabled', 'Enabled'}  vector_style=Wide Row  use_help_units=on  help='Base air request position, includes ramp into idle manager.'  units='%'  use_header_enum=off  row_header_enum={}  col_header_enum={}  use_precision=on  precision='5.2'  gain=1  offset=0  exp=1  use_mototune_group=on  mototune_group=motohawk_vardec_path(gcb)
  BaseAirOffset : Outport
  wires:
  Sensors/1 -> Bus Selector1/1, Bus Selector2/1, Bus Selector3/1
  Bus Selector2/1 -> motohawk_interpolation_1d2/1  "<ECT05Idx>"
  Ramp Air Into Idle State/1(TPSSetpoint) -> BaseAirOffset/1, motohawk_probe1/1
  motohawk_data_read/1 -> Run/1
  Unit Delay/1 -> Relational Operator/2, Relational Operator1/2
  Relational Operator/1 -> Logical Operator/2
  Relational Operator1/1 -> Logical Operator/1
  Run/1 -> Relational Operator/1, Relational Operator1/1, Unit Delay/1
  Logical Operator/1 -> Ramp Air Into Idle State/1(EngineState)
  Bus Selector1/1 -> Ramp Air Into Idle State/3(InitialSetpoint)  "<TPS>"
  motohawk_interpolation_1d2/1 -> Sum/2
  Sum/1 -> Ramp Air Into Idle State/2(TPSOffset)
  Product/1 -> Sum/1
  motohawk_interpolation_1d1/1 -> Product/3
  motohawk_calibration/1 -> Product/1
  AC/1 -> Product/2
  Bus Selector3/1 -> motohawk_interpolation_1d1/1  "<ACPres05Idx>"

== system BaseEngineController_LS/Foreground/Control/Controller/Run/MinGovernor/Base Airflow Table Adapt ==
  Idle State : Inport
  ITerm : Inport  Port=2
  Enable : EnablePort
  Abs : Abs  SaturateOnIntegerOverflow=on
  Adapt Base Airflow Table : Subsystem  TreatAsAtomicUnit=on
  Idle Control Enable Delay : Subsystem  TreatAsAtomicUnit=on
  Logical Operator1 : Logic  Inputs=3
  Product0 : Product  SaturateOnIntegerOverflow=on  InputSameDT=on  OutDataTypeStr=Inherit: Same as first input
  Relational Operator : RelationalOperator  Operator=<=  InputSameDT=on
  Saturation (Tunable) : Subsystem  AncestorBlock=motohawk_control_primitives_lib/Saturation (Tunable)  mask(Saturation (Tunable)){prefix='BaseAirflowAdaptError', UprLim=1, LwrLim=-1, units='', grp=motohawk_vardec_path(gcb)}
      mask prompts: UprLim "Upper Limit"; LwrLim "Lower Limit"; grp "MotoTune Group String"
      mask help: Saturation block with calibratable min/max values.
      mask Display:
      | patch([0 0 1 1], [0 0.075 0.075 0], [230/255 0/255 0/255])
      | patch([0 0 1 1], [0.025 0.05 0.05 0.025], [150/255 0/255 0/255])
      | patch([0 0 1 1], [0 0.025 0.025 0], [0/255 0/255 0/255])
      | 
      | plot([0 .2 .8 1], [.1 .1 1 1])
  motohawk_calibration2 : MotoHawk_lib/Calibration & Probing Blocks/motohawk_calibration  nam='BaseAirflowAdaptGain'  val=0.001  storage=Calibration  show_more=on  name_source=Use Parameter  data_type=Inherit from 'Default Value'  read_level=1  write_level=1  ovr_cals=on  view_as=Number  enum_struct={'Disabled', 'Enabled'}  vector_style=Wide Row  use_help_units=off  help="'Gain for updating BaseAirflow table.  This fraction of the error is added to the map every 5ms.'"  units='mult'  use_header_enum=off  row_header_enum={}  col_header_enum={}  use_min_max=off  min_val=-inf  max_val=inf  use_precision=on  precision='1.4'  gain=1  offset=0  exp=1  use_mototune_group=on  mototune_group=motohawk_vardec_path(gcb)
  motohawk_calibration3 : MotoHawk_lib/Calibration & Probing Blocks/motohawk_calibration  nam='BaseAirflowAdaptDelta'  val=2  storage=Calibration  show_more=on  name_source=Use Parameter  data_type=Inherit from 'Default Value'  read_level=1  write_level=1  ovr_cals=on  view_as=Number  enum_struct={'Disabled', 'Enabled'}  vector_style=Wide Row  use_help_units=on  help='Air PID Iterm must be less than this delta to adapt the BaseAirflow table.'  units='mult'  use_header_enum=off  row_header_enum={}  col_header_enum={}  use_min_max=on  min_val=-inf  max_val=inf  use_precision=off  precision=''  gain=1  offset=0  exp=1  use_mototune_group=on  mototune_group=motohawk_vardec_path(gcb)
  motohawk_calibration4 : MotoHawk_lib/Calibration & Probing Blocks/motohawk_calibration  nam='BaseAirflowAdaptEnable'  val=true  storage=Calibration  show_more=on  name_source=Use Parameter  data_type=Inherit from 'Default Value'  read_level=1  write_level=1  ovr_cals=on  view_as=Enumeration  enum_struct={'Disabled', 'Enabled'}  vector_style=Wide Row  use_help_units=on  help='Determines whether the BaseAirflow table will be adapted using the air PID Iterm.'  units='bool'  use_header_enum=off  row_header_enum={}  col_header_enum={}  use_min_max=off  min_val=-inf  max_val=inf  use_precision=off  precision=''  gain=1  offset=0  exp=1  use_mototune_group=on  mototune_group=motohawk_vardec_path(gcb)
  motohawk_probe3 : MotoHawk_lib/Calibration & Probing Blocks/motohawk_probe  nam='BaseAirflowAdaptEnabled'  show_more=on  name_source=Use Parameter  read_level=1  view_as=Enumeration  enum_struct={'Not Enabled', 'Enabled'}  vector_style=Wide Row  use_help_units=on  help=''  units=''  use_header_enum=off  row_header_enum={}  col_header_enum={}  use_precision=off  precision=''  gain=1  offset=0  exp=1  use_mototune_group=on  mototune_group=motohawk_vardec_path(gcb)
  wires:
  Abs/1 -> Relational Operator/1
  motohawk_calibration3/1 -> Relational Operator/2
  motohawk_calibration2/1 -> Product0/2
  Product0/1 -> Saturation (Tunable)/1(In)
  ITerm/1 -> Product0/1, Abs/1
  Relational Operator/1 -> Logical Operator1/3
  Idle Control Enable Delay/1(State_Out) -> Logical Operator1/2
  Logical Operator1/1 -> motohawk_probe3/1, Adapt Base Airflow Table/Enable
  Saturation (Tunable)/1(Out) -> Adapt Base Airflow Table/1(error)
  motohawk_calibration4/1 -> Logical Operator1/1
  Idle State/1 -> Idle Control Enable Delay/1(State_In)

== system BaseEngineController_LS/Foreground/Control/Controller/Run/MinGovernor/Base RPM Set Pt ==
  Sensors : Inport
  Bus Selector2 : BusSelector  OutputSignals=RawIndexes.ECT05Idx
  motohawk_interpolation_1d2 : MotoHawk_lib/Lookup Tables/motohawk_interpolation_1d  nam='MinGovClntRPMSetPt'  table_data=[1000 990 965 850 650]  show_more=on  data_type=int16  storage=NonAdaptive  read_level=1  write_level=1  ovr_cals=on  use_help=on  help='RPM setpoint based on ECT.'  units='RPM'  use_min_max=on  min_val=-inf  max_val=inf  use_precision=on  precision=''  gain=1  offset=0  exp=1  use_links=off  prelookup_block=''  output_name=''  use_mototune_group=on  mototune_group=motohawk_vardec_path(gcb)
  RPMSetPt : Outport
  wires:
  motohawk_interpolation_1d2/1 -> RPMSetPt/1
  Bus Selector2/1 -> motohawk_interpolation_1d2/1  "<ECT05Idx>"
  Sensors/1 -> Bus Selector2/1
